simulink model "sim_cv_3"  (R2025b)
settings: Solver=VariableStepAuto  StartTime=0.0  StopTime=1200  RelTol=1e-3
values from neighbouring files (symbols this model uses):
  inv_S1 = 1 / S1    (= 1)    [cv_3.m]
  inv_S2 = 1 / S2    (= 1)    [cv_3.m]
  K_out1 = mu * S10 * sqrt(2 * g)    [cv_3.m]
  K_out2 = mu * S20 * sqrt(2 * g)    [cv_3.m]
  Q1_final = Q1_initial / 2    (= 0.00971)    [cv_3.m]
  Q1_initial = 0.01942    [cv_3.m]
  Q1_step_time = 700    [cv_3.m]
  Q1_target_sys1 = mu * S20 * sqrt(2 * g * h2_target)    [cv_3.m]
  Q1_target_sys2 = (mu * S10 * sqrt(2) + mu * S20) * sqrt(2 * g * h2_target)    [cv_3.m]
settings Model: Creator=yehor  LastModifiedBy=yehor

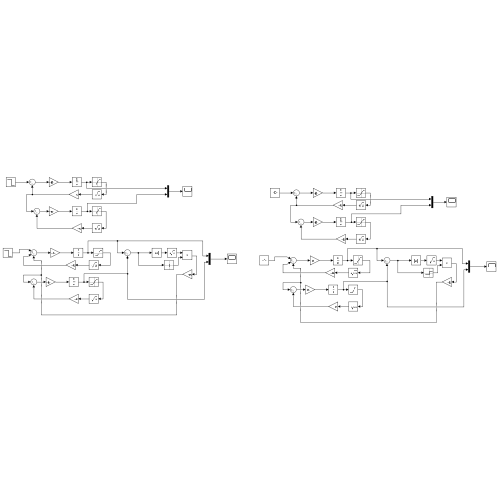
[thumbnail: Simulink's stored preview of the top-level diagram]
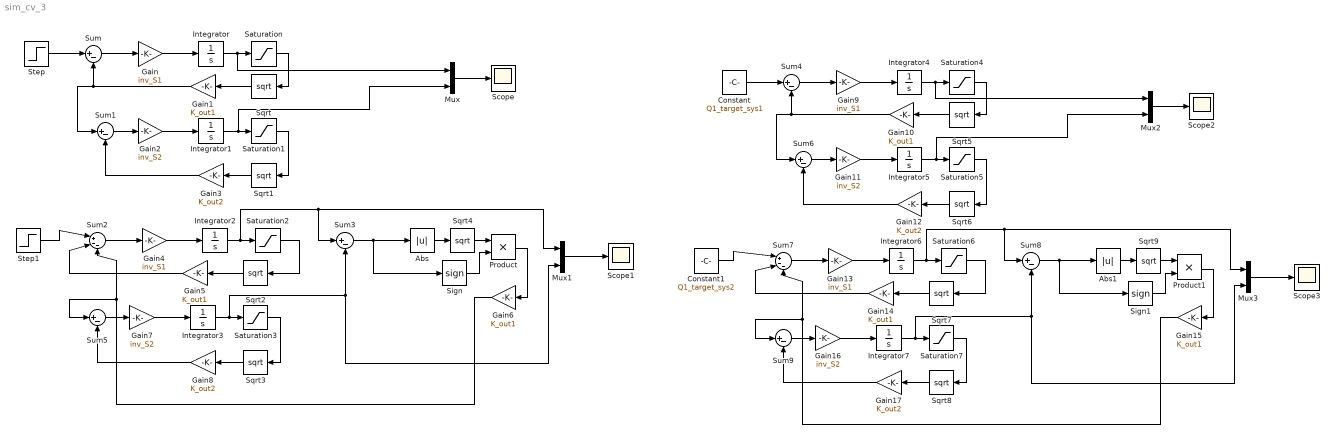
== system sim_cv_3 ==
  Abs : Abs  SaturateOnIntegerOverflow=off
  Abs1 : Abs  SaturateOnIntegerOverflow=off
  Constant : Constant  Value=Q1_target_sys1
  Constant1 : Constant  Value=Q1_target_sys2
  Gain{,4,9,13} (4 alike) : Gain  Gain=inv_S1
  Gain{1,5..6,10,14..15} (6 alike) : Gain  Gain=K_out1
  Gain{2,7,11,16} (4 alike) : Gain  Gain=inv_S2
  Gain{3,8,12,17} (4 alike) : Gain  Gain=K_out2
  Integrator{,1..7} (8 alike) : Integrator
  Mux{,1..3} (4 alike) : Mux  Inputs=2
  Product : Product
  Product1 : Product
  Saturation{,1..7} (8 alike) : Saturate  UpperLimit=inf  LowerLimit=0
  Scope{,1..3} (4 alike) : Scope
      Scope settings: ActiveDisplayYMinimum=-0.13520215592759616  ActiveDisplayYMaximum=0.62666498492923206
      Scope1 settings: ActiveDisplayYMinimum=-1  ActiveDisplayYMaximum=1
      Scope2 settings: ActiveDisplayYMinimum=-0.02657455338657  ActiveDisplayYMaximum=0.52660652169727451  DataLoggingVariableName=ScopeData2
      Scope3 settings: ActiveDisplayYMinimum=-0.35718056358015315  ActiveDisplayYMaximum=0.94085006190097775  DataLoggingVariableName=ScopeData3
  Sign : Signum
  Sign1 : Signum
  Sqrt{,1..9} (10 alike) : Sqrt
  Step : Step  Time=Q1_step_time  Before=Q1_initial  After=Q1_final  SampleTime=0
  Step1 : Step  Time=Q1_step_time  Before=Q1_initial  After=Q1_final  SampleTime=0
  Sum{,1,3..6,8..9} (8 alike) : Sum  Inputs=|+-
  Sum2 : Sum  Inputs=|+--
  Sum7 : Sum  Inputs=|+--
  wires:
  Step/1 -> Sum/1
  Sum/1 -> Gain/1
  Gain/1 -> Integrator/1
  Integrator/1 -> Mux/1, Saturation/1
  Saturation/1 -> Sqrt/1
  Sqrt/1 -> Gain1/1
  Gain1/1 -> Sum1/1, Sum/2
  Sum1/1 -> Gain2/1
  Gain2/1 -> Integrator1/1
  Integrator1/1 -> Mux/2, Saturation1/1
  Saturation1/1 -> Sqrt1/1
  Sqrt1/1 -> Gain3/1
  Gain3/1 -> Sum1/2
  Mux/1 -> Scope/1
  Sum3/1 -> Sign/1, Abs/1
  Abs/1 -> Sqrt4/1
  Sign/1 -> Product/2
  Product/1 -> Gain6/1
  Gain6/1 -> Sum5/1, Sum2/3
  Saturation3/1 -> Sqrt3/1
  Saturation2/1 -> Sqrt2/1
  Sqrt2/1 -> Gain5/1
  Step1/1 -> Sum2/1
  Integrator2/1 -> Mux1/1, Sum3/1, Saturation2/1
  Sum2/1 -> Gain4/1
  Gain7/1 -> Integrator3/1
  Gain4/1 -> Integrator2/1
  Integrator3/1 -> Sum3/2, Mux1/2, Saturation3/1
  Gain5/1 -> Sum2/2
  Sqrt3/1 -> Gain8/1
  Sum5/1 -> Gain7/1
  Gain8/1 -> Sum5/2
  Sqrt4/1 -> Product/1
  Mux1/1 -> Scope1/1
  Saturation5/1 -> Sqrt6/1
  Saturation4/1 -> Sqrt5/1
  Sqrt5/1 -> Gain10/1
  Constant/1 -> Sum4/1
  Mux2/1 -> Scope2/1
  Sum4/1 -> Gain9/1
  Gain11/1 -> Integrator5/1
  Gain9/1 -> Integrator4/1
  Integrator4/1 -> Mux2/1, Saturation4/1
  Integrator5/1 -> Mux2/2, Saturation5/1
  Gain10/1 -> Sum6/1, Sum4/2
  Sqrt6/1 -> Gain12/1
  Sum6/1 -> Gain11/1
  Gain12/1 -> Sum6/2
  Constant1/1 -> Sum7/1
  Saturation6/1 -> Sqrt7/1
  Saturation7/1 -> Sqrt8/1
  Gain17/1 -> Sum9/2
  Integrator7/1 -> Sum8/2, Mux3/2, Saturation7/1
  Gain14/1 -> Sum7/2
  Product1/1 -> Gain15/1
  Gain15/1 -> Sum9/1, Sum7/3
  Gain13/1 -> Integrator6/1
  Sum9/1 -> Gain16/1
  Gain16/1 -> Integrator7/1
  Sqrt9/1 -> Product1/1
  Sum8/1 -> Sign1/1, Abs1/1
  Sum7/1 -> Gain13/1
  Abs1/1 -> Sqrt9/1
  Sign1/1 -> Product1/2
  Sqrt8/1 -> Gain17/1
  Sqrt7/1 -> Gain14/1
  Integrator6/1 -> Mux3/1, Sum8/1, Saturation6/1
  Mux3/1 -> Scope3/1
